simulink model "HW2_Q4_P3"  (R2018b)
settings: Solver=VariableStepAuto  StartTime=0.0  StopTime=150.0  RelTol=1e-3
settings Model: Creator=mohammadreza  LastModifiedBy=mohammadreza

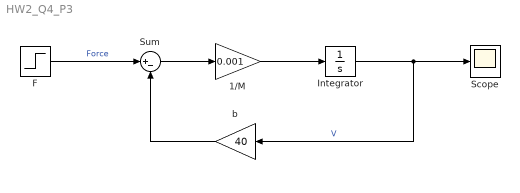
== system HW2_Q4_P3 ==
  1/M : Gain  Gain=0.001
  F : Step  Time=0  After=500  SampleTime=0
  Integrator : Integrator
  Scope : Scope
  Sum : Sum  Inputs=|+-
  b : Gain  Gain=40
  wires:
  b/1 -> Sum/2
  F/1 -> Sum/1  "Force"
  Sum/1 -> 1/M/1
  1/M/1 -> Integrator/1
  Integrator/1 -> b/1, Scope/1  "V"
